simulink model "fw_pos_control"  (R2021a)
settings: Solver=FixedStepAuto  StartTime=0.0  StopTime=5  FixedStep=0.02  RelTol=1e-3
undefined symbols (not defined in the file): DiscIntNeverNeededParam, DT_DEFAULT, FW_AIRSPD_MAX, FW_AIRSPD_MIN, FW_L1_DAMPING, FW_L1_PERIOD, FW_L1_R_SLEW_MAX, FW_R_LIM, FW_T_CLMB_MAX, FW_T_HRATE_FF, FW_T_I_GAIN_PIT, FW_T_I_GAIN_THR, FW_T_PTCH_DAMP, FW_T_RLL2THR, FW_T_SEB_R_FF, FW_T_SINK_MAX, FW_T_SINK_MIN, FW_T_SPD_OMEGA, FW_T_STE_R_TC, FW_T_TAS_TC, FW_T_THR_DAMP, FW_T_VERT_ACC, FW_THR_CRUISE, FW_THR_MAX, FW_THR_MIN, FW_THR_SLEW_MAX, GRAVITY, magnitude
libraries: simulink x28, vrlib x3
(part 3 of 4)

== stateflow chart fw_pos_control/FW Control ==
  state rotary_wing
    en,du:
    sprintf("current sample time is %f", getSimulationTime);
  state fixed_wing
    en,du:
    % 定义中间变量
    fixed_wing.define_variables;
    % 轮询相关数据
    [airspeed_valid_, eas2tas_] = fixed_wing.airspeed_poll;
    [man_ctr_sp_alt_, man_ctr_sp_aspd_] = fixed_wing.manual_control_setpoint_poll;
    [yaw_, pitch_, roll_] = fixed_wing.vehicle_attitude_poll;
    [last_manual_] = fixed_wing.vehicle_control_mode_poll;
    [nav_speed_2d_, ground_speed_2d_] = fixed_wing.vehicle_update_nav_speed;
    % 默认不直接控制方向舵，不使用襟翼，油门不限幅
    out_att_sp.fw_control_yaw = false;
    out_att_sp.apply_flaps = uint8(PX4_VEHICLE_ATTITUDE_SETPOINT.FLAPS_OFF);
    throttle_max_ = 1.0;
    state onGround_or_inTakeoffSituation [parallel]
      settings: executionOrder=1
      state on_ground
        en:
        was_in_air_ = false;
      state in_takeOffSituation
        en:
        %记录起飞时间和起飞高度
        was_in_air_ = true;
        time_went_in_air_ = uint64(getSimulationTime);
        takeoff_ground_alt_ = current_alt_;
        en, du:
        in_takeoff_situation_ = is_takeoff_situation;
      (default) -> on_ground
      on_ground -> in_takeOffSituation : %上一时刻在地上，当前时刻在空中
          | [~was_in_air_ && ~landed_]
      in_takeOffSituation -> on_ground : [landed_]
    state position_control [parallel]
      settings: executionOrder=2
      state mode_select [parallel]
        settings: executionOrder=1
        (default) -> (junction 1468)
        mode_select -> (junction 1468)
        (junction 1468) -> (junction 1469) [order 1] : [control_mode.flag_control_auto_enabled || control_mode.flag_control_offboard_enabled]
        (junction 1468) -> (junction 1470) [order 2]
        (junction 1469) -> (junction 1477) : {pos_control_mode_ = PX4_FW_CONTROL.AUTO_MODE;}
        (junction 1470) -> (junction 1471) [order 1] : [control_mode.flag_control_velocity_enabled && control_mode.flag_control_altitude_enabled]
        (junction 1470) -> (junction 1472) [order 2]
        (junction 1471) -> (junction 1476) : {pos_control_mode_ = PX4_FW_CONTROL.POS_MODE;}
        (junction 1472) -> (junction 1473) [order 1] : [control_mode.flag_control_altitude_enabled]
        (junction 1472) -> (junction 1474) [order 2] : {pos_control_mode_ = PX4_FW_CONTROL.OTHER_MODE;}
        (junction 1473) -> (junction 1475) : {pos_control_mode_ = PX4_FW_CONTROL.ALT_MODE;}
        (junction 1475) -> (junction 1474)
        (junction 1476) -> (junction 1475)
        (junction 1477) -> (junction 1476)
        (junction 1474) -> (junction 1478)
      state mode_action [parallel]
        settings: executionOrder=2
        state auto_offboard_mode [parallel]
          settings: executionOrder=1
          state not_run
            en,du:
          state running
            en,du:
            is_transition_to_fw;
            state auto_logical [parallel]
              settings: executionOrder=1
              (default) -> (junction 2990)
              (junction 2990) -> (junction 2989) [order 1] : [(curr_wp_type_ == PX4_POSITION_SETPOINT.SETPOINT_TYPE_TAKEOFF) && ...
                  |  (~in_takeoff_situation_) && ...
                  |  (airspeed_validated.calibrated_airspeed_m_s >= FW_AIRSPD_MIN)]
              auto_logical -> (junction 2990) : {curr_wp_type_ = uint8(pos_sp_curr_.type);
                  | [dist_xy, dist_z, dist] = get_distance_to_point_global_wgs84(pos_sp_curr_.lat, pos_sp_curr_.lon, pos_sp_curr_.alt, ...
                  |     current_lat_, current_lon_, current_alt_);}
              (junction 2989) -> (junction 2996) : {curr_wp_type_ = uint8(PX4_POSITION_SETPOINT.SETPOINT_TYPE_POSITION);}
              (junction 2990) -> (junction 2992) [order 2]
              (junction 2992) -> (junction 2991) [order 1] : % 飞机还没有越过当前航点，且当前的高度大于2倍FW_CLMBOUT_DIFF，
                  | % 但是水平距离小于2倍可接受的距离以内，飞机改为盘旋的方式靠近当前航点
                  | % FW_CLMBOUT_DIFF 默认10m
                  | [(curr_wp_type_ == PX4_POSITION_SETPOINT.SETPOINT_TYPE_POSITION) && ...
                  |  (dist > 0.0) && ...
                  |  (dist > 2.0 * FW_CLMBOUT_DIFF) && ...
                  |  (dist_xy < 2.0 * max(acc_rad, abs(pos_sp_triplet.current.loiter_radius)))]
              (junction 2991) -> (junction 2995) : {curr_wp_type_ == uint8(PX4_POSITION_SETPOINT.SETPOINT_TYPE_LOITER);}
              (junction 2992) -> (junction 2993) [order 2]
              (junction 2993) -> (junction 2994) [order 1] : % 飞机还没有越过当前航点，且当前的高度大于2倍FW_CLMBOUT_DIFF，
                  | % 同时水平距离也大于2倍可接受的距离以外，飞机继续以position的方式靠近当前航点
                  | % FW_CLMBOUT_DIFF 默认10m
                  | [(curr_wp_type_ == PX4_POSITION_SETPOINT.SETPOINT_TYPE_LOITER) && ...
                  |  (dist > 0.0) && ...
                  |  (dist > 2.0 * FW_CLMBOUT_DIFF) && ...
                  |  (dist_xy < 2.0 * max(acc_rad, max(acc_rad, pos_sp_triplet.current.loiter_radius)))]
              (junction 2993) -> (junction 2997) [order 2]
              (junction 2994) -> (junction 2998) : {curr_wp_type_ == uint8(PX4_POSITION_SETPOINT.SETPOINT_TYPE_POSITION);}
              (junction 2996) -> (junction 2995)
              (junction 2995) -> (junction 2998)
              (junction 2998) -> (junction 2997)
              (junction 2997) -> (junction 2999)
            state auto_action [parallel]
              settings: executionOrder=2
              state idle [parallel]
                settings: executionOrder=1
                state not_run
                  en,du:
                state running
                  en,du:
                  reset_landing_state;
                  reset_takeoff_state(false);
                  out_att_sp.roll_body = single(0.0);
                  out_att_sp.pitch_body = single(deg2rad(FW_PSP_OFF));
                  out_att_sp.thrust_body(1)  = single(0.0);
                  if (was_circle_mode_ && ~circle_mode_)
                  out_att_sp.roll_reset_integral = true;
                  else
                  out_att_sp.roll_reset_integral = false;
                  end
                (default) -> fixed_wing.position_control.mode_action.auto_offboard_mode.running.auto_action.idle.not_run
                fixed_wing.position_control.mode_action.auto_offboard_mode.running.auto_action.idle.not_run -> fixed_wing.position_control.mode_action.auto_offboard_mode.running.auto_action.idle.running : [curr_wp_type_ == uint8(PX4_POSITION_SETPOINT.SETPOINT_TYPE_IDLE)]
                fixed_wing.position_control.mode_action.auto_offboard_mode.running.auto_action.idle.running -> fixed_wing.position_control.mode_action.auto_offboard_mode.running.auto_action.idle.not_run : [curr_wp_type_ ~= uint8(PX4_POSITION_SETPOINT.SETPOINT_TYPE_IDLE)]
              state position [parallel]
                settings: executionOrder=2
                state not_run
                  en,du:
                state running
                  en,du:
                  position_sp_alt = get_foh_alt;
                  % l1控制, 输出att_sp.roll-body, att_sp.yaw_body
                  [out_att_sp.roll_body, out_att_sp.yaw_body, ...
                  l1_target_bearing_, l1_crosstrack_error_, ...
                  l1_distance_, circle_mode_] = ...
                  mode_action.l1_navigate_waypoints(prev_wp_, curr_wp_, curr_pos_, nav_speed_2d_, out_att_sp.roll_body);
                  % tecs控制
                  [run_tecs_, tecs_input_] = mode_action.prepare_tecs_controller_param(position_sp_alt, ...
                  fixed_wing.cal_target_aspd(mission_airspeed_), ...
                  deg2rad(FW_P_LIM_MIN), ...
                  deg2rad(FW_P_LIM_MAX), ...
                  tecs_fw_thr_min, ...
                  tecs_fw_thr_max, ...
                  tecs_fw_mission_throttle, ...
                  false, ...
                  deg2rad(FW_P_LIM_MIN), ...
                  PX4_TECS_STATUS.TECS_MODE_NORMAL, ...
                  nan);
                  % 输出att_sp.pitch_body, roll_reset_integral, thrust_body
                  if (run_tecs_ == true)
                  [tecs_throttle_sp_, tecs_pitch_sp_, tecs_hgt_rate_sp_, tecs_mode_] = mode_action.tecs_controller(tecs_input_);
                  out_att_sp.pitch_body = single(tecs_pitch_sp_ + deg2rad(FW_PSP_OFF));
                  else
                  out_att_sp.pitch_body = single(deg2rad(FW_PSP_OFF));
                  end
                  fixed_wing.reset_landing_state;
                  fixed_wing.reset_takeoff_state(false);
                  if (was_circle_mode_ && ~circle_mode_)
                  out_att_sp.roll_reset_integral = true;
                  else
                  out_att_sp.roll_reset_integral = false;
                  end
                  out_att_sp.thrust_body(1) = constrain(tecs_throttle_sp_, 0.0, 1.0);
                (default) -> fixed_wing.position_control.mode_action.auto_offboard_mode.running.auto_action.position.not_run
                fixed_wing.position_control.mode_action.auto_offboard_mode.running.auto_action.position.not_run -> fixed_wing.position_control.mode_action.auto_offboard_mode.running.auto_action.position.running : [curr_wp_type_ == uint8(PX4_POSITION_SETPOINT.SETPOINT_TYPE_POSITION)]
                fixed_wing.position_control.mode_action.auto_offboard_mode.running.auto_action.position.running -> fixed_wing.position_control.mode_action.auto_offboard_mode.running.auto_action.position.not_run : [curr_wp_type_ ~= uint8(PX4_POSITION_SETPOINT.SETPOINT_TYPE_POSITION)]
              state loiter [parallel]
                settings: executionOrder=3
                state not_run
                  en,du:
                state running
                  en,du:
                  [out_att_sp.roll_body, out_att_sp.yaw_body, l1_target_bearing_, l1_distance_, circle_mode_] = ...
                  mode_action.l1_navigate_loiter(curr_wp_, curr_pos_, ...
                  pos_sp_curr_.loiter_direction, nav_speed_2d_, ...
                  pos_sp_curr_.loiter_radius, circle_mode_, out_att_sp.roll_body);
                  state loiter_logical [parallel]
                    settings: executionOrder=1
                    (default) -> (junction 3043)
                    (junction 3043) -> (junction 3044) [order 1] : [pos_sp_triplet.next.type == PX4_POSITION_SETPOINT.SETPOINT_TYPE_LAND && ...
                        | pos_sp_triplet.next.valid && ...
                        | circle_mode_ && ...
                        | FW_LND_EARLYCFG]
                    (junction 3043) -> (junction 3045) [order 2]
                    (junction 3044) -> (junction 3052) : {loiter_type_ = PX4_LOITER_TYPE.NEXT_WP_LAND}
                    (junction 3045) -> (junction 3046) [order 1] : [in_takeoff_situation_]
                    (junction 3045) -> (junction 3047) [order 2]
                    (junction 3046) -> (junction 3051) : {loiter_type_ = PX4_LOITER_TYPE.IN_TAKEOFF_SITUATION}
                    (junction 3047) -> (junction 3048) [order 1] : [land_abort_]
                    (junction 3047) -> (junction 3049) [order 2] : {loiter_type_ = PX4_LOITER_TYPE.DEFAULT}
                    (junction 3048) -> (junction 3050) : {loiter_type_ = PX4_LOITER_TYPE.LAND_ABORT}
                    (junction 3050) -> (junction 3049)
                    (junction 3051) -> (junction 3050)
                    (junction 3052) -> (junction 3051)
                    (junction 3049) -> (junction 3053)
                  state loiter_action [parallel]
                    settings: executionOrder=2
                    state next_wp_land [parallel]
                      settings: executionOrder=1
                      state not_run
                        en,du:
                      state running
                        en,du:
                        tecs_height_error_gain_ = single(1.0 / max(FW_LND_THRTC_SC * FW_T_ALT_TC, 0.1));
                        out_att_sp.apply_flaps = uint8(PX4_VEHICLE_ATTITUDE_SETPOINT.FLAPS_LAND);
                        [run_tecs_, tecs_input_] = mode_action.prepare_tecs_controller_param(pos_sp_curr_.alt, ...
                        fixed_wing.cal_target_aspd(FW_LND_AIRSPD_SC * FW_AIRSPD_MIN), ...
                        deg2rad(FW_P_LIM_MIN), ...
                        deg2rad(FW_P_LIM_MAX), ...
                        tecs_fw_thr_min, ...
                        tecs_fw_thr_max, ...
                        tecs_fw_mission_throttle, ...
                        false, ...
                        deg2rad(FW_P_LIM_MIN), ...
                        PX4_TECS_STATUS.TECS_MODE_NORMAL, ...
                        nan);
                        if (run_tecs_ == true)
                        [tecs_throttle_sp_, tecs_pitch_sp_, tecs_hgt_rate_sp_, tecs_mode_] = ...
                        mode_action.tecs_controller(tecs_input_);
                        out_att_sp.pitch_body = single(tecs_pitch_sp_ + deg2rad(FW_PSP_OFF));
                        else
                        out_att_sp.pitch_body = single(deg2rad(FW_PSP_OFF));
                        end
                        fixed_wing.reset_landing_state;
                        fixed_wing.reset_takeoff_state(false);
                        if (was_circle_mode_ && ~circle_mode_)
                        out_att_sp.roll_reset_integral = true;
                        else
                        out_att_sp.roll_reset_integral = true;
                        end
                        out_att_sp.thrust_body(1) = tecs_throttle_sp_;
                      (default) -> fixed_wing.position_control.mode_action.auto_offboard_mode.running.auto_action.loiter.running.loiter_action.next_wp_land.not_run
                      fixed_wing.position_control.mode_action.auto_offboard_mode.running.auto_action.loiter.running.loiter_action.next_wp_land.not_run -> fixed_wing.position_control.mode_action.auto_offboard_mode.running.auto_action.loiter.running.loiter_action.next_wp_land.running : [loiter_type_ == PX4_LOITER_TYPE.NEXT_WP_LAND]
                      fixed_wing.position_control.mode_action.auto_offboard_mode.running.auto_action.loiter.running.loiter_action.next_wp_land.running -> fixed_wing.position_control.mode_action.auto_offboard_mode.running.auto_action.loiter.running.loiter_action.next_wp_land.not_run : [loiter_type_ ~= PX4_LOITER_TYPE.NEXT_WP_LAND]
                    state in_takeoff_situation [parallel]
                      settings: executionOrder=2
                      state runing
                        en,du:
                        out_att_sp.roll_body = constrain(out_att_sp.roll_body, deg2rad(-5.0), deg2rad(5.0));
                        [run_tecs_, tecs_input_] = mode_action.prepare_tecs_controller_param(...
                        max(pos_sp_curr_.alt, takeoff_ground_alt_ + FW_CLMBOUT_DIFF), ...
                        cal_target_aspd(mission_airspeed_), ...
                        deg2rad(FW_P_LIM_MIN), ...
                        deg2rad(FW_P_LIM_MAX), ...
                        tecs_fw_thr_min, ...
                        tecs_fw_thr_max, ...
                        tecs_fw_mission_throttle, ...
                        false, ...
                        deg2rad(FW_P_LIM_MIN), ...
                        PX4_TECS_STATUS.TECS_MODE_NORMAL, ...
                        nan);
                        if (run_tecs_ == true)
                        [tecs_throttle_sp_, tecs_pitch_sp_, tecs_hgt_rate_sp_, tecs_mode_] = tecs_controller(tecs_input_);
                        out_att_sp.pitch_body = single(tecs_pitch_sp_ + deg2rad(FW_PSP_OFF));
                        else
                        out_att_sp.pitch_body = single(deg2rad(FW_PSP_OFF));
                        end
                        fixed_wing.reset_landing_state;
                        fixed_wing.reset_takeoff_state(false);
                        if (was_circle_mode_ && ~circle_mode_)
                        out_att_sp.roll_reset_integral = true;
                        end
                        out_att_sp.thrust_body(1) = tecs_throttle_sp_;
                      state not_run
                        en,du:
                      (default) -> fixed_wing.position_control.mode_action.auto_offboard_mode.running.auto_action.loiter.running.loiter_action.in_takeoff_situation.not_run
                      fixed_wing.position_control.mode_action.auto_offboard_mode.running.auto_action.loiter.running.loiter_action.in_takeoff_situation.not_run -> runing : [loiter_type_ == PX4_LOITER_TYPE.IN_TAKEOFF_SITUATION]
                      runing -> fixed_wing.position_control.mode_action.auto_offboard_mode.running.auto_action.loiter.running.loiter_action.in_takeoff_situation.not_run : [loiter_type_ ~= PX4_LOITER_TYPE.IN_TAKEOFF_SITUATION]
                    state land_abort [parallel]
                      settings: executionOrder=3
                      state running
                        en,du:
                        % aborted landing complete, normal loiter over landing point
                        if (pos_sp_curr_.alt - current_alt_ < FW_CLMBOUT_DIFF)
                        land_abort_ = false;
                        else
                        % continue straight until vehicle has sufficient altitude
                        out_att_sp.roll_body = single(0.0);
                        end
                        tecs_height_error_gain_ = single(1.0 / max(FW_LND_THRTC_SC * FW_T_ALT_TC, 0.1));
                        [run_tecs_, tecs_input_] = mode_action.prepare_tecs_controller_param(pos_sp_curr_.alt, ...
                        cal_target_aspd(mission_airspeed_), ...
                        deg2rad(FW_P_LIM_MIN), ...
                        deg2rad(FW_P_LIM_MAX), ...
                        tecs_fw_thr_min, ...
                        tecs_fw_thr_max, ...
                        tecs_fw_mission_throttle, ...
                        false, ...
                        deg2rad(FW_P_LIM_MIN), ...
                        PX4_TECS_STATUS.TECS_MODE_NORMAL, ...
                        nan);
                        if (run_tecs_ == true)
                        [tecs_throttle_sp_, tecs_pitch_sp_, tecs_hgt_rate_sp_, tecs_mode_] = mode_action.tecs_controller(tecs_input_);
                        out_att_sp.pitch_body = single(tecs_pitch_sp_ + deg2rad(FW_PSP_OFF));
                        else
                        out_att_sp.pitch_body = single(deg2rad(FW_PSP_OFF));
                        end
                        fixed_wing.reset_landing_state;
                        fixed_wing.reset_takeoff_state(false);
                        if (was_circle_mode_ && ~circle_mode_)
                        out_att_sp.roll_reset_integral = true;
                        else
                        out_att_sp.roll_reset_integral = false;
                        end
                        out_att_sp.thrust_body(1) = tecs_throttle_sp_;
                      state not_run
                        en,du:
                      (default) -> fixed_wing.position_control.mode_action.auto_offboard_mode.running.auto_action.loiter.running.loiter_action.land_abort.not_run
                      fixed_wing.position_control.mode_action.auto_offboard_mode.running.auto_action.loiter.running.loiter_action.land_abort.not_run -> fixed_wing.position_control.mode_action.auto_offboard_mode.running.auto_action.loiter.running.loiter_action.land_abort.running : [loiter_type_ == PX4_LOITER_TYPE.LAND_ABORT]
                      fixed_wing.position_control.mode_action.auto_offboard_mode.running.auto_action.loiter.running.loiter_action.land_abort.running -> fixed_wing.position_control.mode_action.auto_offboard_mode.running.auto_action.loiter.running.loiter_action.land_abort.not_run : [loiter_type_ ~= PX4_LOITER_TYPE.LAND_ABORT]
                    state default [parallel]
                      settings: executionOrder=4
                      state not_run
                        en,du:
                      state running
                        en,du:
                        [run_tecs_, tecs_input_] = mode_action.prepare_tecs_controller_param(pos_sp_curr_.alt, ...
                        airspeed_demand_, ...
                        deg2rad(FW_P_LIM_MIN), ...
                        deg2rad(FW_P_LIM_MAX), ...
                        tecs_fw_thr_min, ...
                        tecs_fw_thr_max, ...
                        tecs_fw_mission_throttle, ...
                        false, ...
                        deg2rad(FW_P_LIM_MIN), ...
                        PX4_TECS_STATUS.TECS_MODE_NORMAL, ...
                        nan);
                        if (run_tecs_ == true)
                        [tecs_throttle_sp_, tecs_pitch_sp_, tecs_hgt_rate_sp_, tecs_mode_] = mode_action.tecs_controller(tecs_input_);
                        out_att_sp.pitch_body = single(tecs_pitch_sp_ + deg2rad(FW_PSP_OFF));
                        else
                        out_att_sp.pitch_body = single(deg2rad(FW_PSP_OFF));
                        end
                        fixed_wing.reset_landing_state;
                        fixed_wing.reset_takeoff_state(false);
                        if (was_circle_mode_ && ~circle_mode_)
                        out_att_sp.roll_reset_integral = true;
                        else
                        out_att_sp.roll_reset_integral = false;
                        end
                        out_att_sp.thrust_body(1) = tecs_throttle_sp_;
                      (default) -> fixed_wing.position_control.mode_action.auto_offboard_mode.running.auto_action.loiter.running.loiter_action.default.not_run
                      fixed_wing.position_control.mode_action.auto_offboard_mode.running.auto_action.loiter.running.loiter_action.default.not_run -> fixed_wing.position_control.mode_action.auto_offboard_mode.running.auto_action.loiter.running.loiter_action.default.running : [loiter_type_ == PX4_LOITER_TYPE.DEFAULT]
                      fixed_wing.position_control.mode_action.auto_offboard_mode.running.auto_action.loiter.running.loiter_action.default.running -> fixed_wing.position_control.mode_action.auto_offboard_mode.running.auto_action.loiter.running.loiter_action.default.not_run : [loiter_type_ ~= PX4_LOITER_TYPE.DEFAULT]
                (default) -> fixed_wing.position_control.mode_action.auto_offboard_mode.running.auto_action.loiter.not_run
                fixed_wing.position_control.mode_action.auto_offboard_mode.running.auto_action.loiter.not_run -> fixed_wing.position_control.mode_action.auto_offboard_mode.running.auto_action.loiter.running : [curr_wp_type_ == uint8(PX4_POSITION_SETPOINT.SETPOINT_TYPE_LOITER)]
                fixed_wing.position_control.mode_action.auto_offboard_mode.running.auto_action.loiter.running -> fixed_wing.position_control.mode_action.auto_offboard_mode.running.auto_action.loiter.not_run : [curr_wp_type_ ~= uint8(PX4_POSITION_SETPOINT.SETPOINT_TYPE_LOITER)]
              state landing [parallel]
                settings: executionOrder=4
                state not_run
                  en,du:
                state running
                  en:
                  fixed_wing.reset_landing_state;
                  time_started_landing_ = uint64(getSimulationTime);
                  en,du:
                  control_landing;
                  land_terrain_alt_ = pos_sp_curr_.alt;
                  out_att_sp.apply_flaps = uint8(PX4_VEHICLE_ATTITUDE_SETPOINT.FLAPS_LAND);
                  state horizontal_control [parallel]
                    settings: executionOrder=1
                    state normal_navigation
                      en,du:
                      [out_att_sp.roll_body, out_att_sp.yaw_body, ...
                      l1_target_bearing_, l1_crosstrack_error_, ...
                      l1_distance_, circle_mode_] = ...
                      mode_action.l1_navigate_waypoints(prev_wp_, ...
                      curr_wp_, curr_pos_, ...
                      nav_speed_2d_, ...
                      out_att_sp.roll_body);
                    state heading_hold
                      en,du:
                      if (pos_sp_prev_.valid)
                      target_bearing_ = bearing_lastwp_currwp_;
                      else
                      target_bearing_ = yaw_;
                      end
                      land_noreturn_horizontal_ = true;
                      [out_att_sp.roll_body, circle_mode_, l1_distance_] = ...
                      mode_action.l1_navigate_heading(target_bearing_, yaw_, ...
                      nav_speed_2d_, out_att_sp.roll_body);
                      out_att_sp.roll_body = constrain(out_att_sp.roll_body, ...
                      deg2rad(10.0), deg2rad(-10.0));
                    (default) -> normal_navigation
                    normal_navigation -> heading_hold : % FW_LND_HHDIST: Landing heading hold horizontal distance, 15m
                        | [(FW_LND_HHDIST > 0.0) && ...
                        |  (~land_noreturn_horizontal_) &&...
                        |  (wp_distance_ < FW_LND_HHDIST) || ...
                        |  (land_noreturn_vertical_)]
                  state vertical_control [parallel]
                    settings: executionOrder=2
                    state glide_slope
                      en,du:
                      [run_tecs_, tecs_input_] = mode_action.prepare_tecs_controller_param(glide_slope, ...
                      cal_target_aspd(FW_LND_AIRSPD_SC * FW_AIRSPD_MIN), ...
                      deg2rad(FW_P_LIM_MIN), ...
                      deg2rad(FW_P_LIM_MAX), ...
                      FW_THR_MIN, ...
                      FW_THR_MAX, ...
                      FW_THR_CRUISE, ...
                      false, ...
                      deg2rad(FW_P_LIM_MIN), ...
                      PX4_TECS_STATUS.TECS_MODE_NORMAL, ...
                      nan);
                      if (run_tecs_ == true)
                      [tecs_throttle_sp_, tecs_pitch_sp_, tecs_hgt_rate_sp_, tecs_mode_] = tecs_controller(tecs_input_);
                      out_att_sp.pitch_body = single(tecs_pitch_sp_ + deg2rad(FW_PSP_OFF));
                      else
                      out_att_sp.pitch_body = single(deg2rad(FW_PSP_OFF));
                      end
                      fixed_wing.reset_takeoff_state(false);
                      if (was_circle_mode_ && ~circle_mode_)
                      out_att_sp.roll_reset_integral = true;
                      end
                    state start_flaring
                      en,du:
                      [land_tecs_mode, land_climbout_pitch_min_rad] = start_flaring;
                      [run_tecs_, tecs_input_] = mode_action.prepare_tecs_controller_param(land_terrain_alt_, ...
                      cal_target_aspd(FW_LND_AIRSPD_SC * FW_AIRSPD_MIN), ...
                      deg2rad(FW_P_LIM_MIN), ...
                      deg2rad(FW_P_LIM_MAX), ...
                      tecs_fw_thr_min, ...
                      tecs_fw_thr_max, ...
                      tecs_fw_mission_throttle, ...
                      false, ...
                      land_climbout_pitch_min_rad, ...
                      land_tecs_mode, ...
                      nan);
                      if (run_tecs_ == true)
                      [tecs_throttle_sp_, tecs_pitch_sp_, tecs_hgt_rate_sp_, tecs_mode_] = tecs_controller(tecs_input_);
                      out_att_sp.pitch_body = single(tecs_pitch_sp_ + deg2rad(FW_PSP_OFF));
                      else
                      out_att_sp.pitch_body = single(deg2rad(FW_PSP_OFF));
                      end
                      if (~land_noreturn_vertical_)
                      % 进入拉平阶段
                      flare_pitch_sp = single(deg2rad(FW_PSP_OFF));
                      flare_height = current_alt_ - land_terrain_alt_;
                      land_noreturn_vertical_ = true;
                      elseif (local_pos.vz > 0.1)
                      % otherwise continue using previous _flare_pitch_sp
                      flare_pitch_sp = single(deg2rad(FW_LND_FL_PMIN) * ...
                      constrain((flare_height - (current_alt_ - land_terrain_alt_)) / flare_height, 0.0, 1.0));
                      end
                      out_att_sp.pitch_body   = flare_pitch_sp;
                      flare_curve_alt_rel_last = flare_curve_alt_rel;
                      fixed_wing.reset_takeoff_state(false);
                      if (was_circle_mode_ && ~circle_mode_)
                      out_att_sp.roll_reset_integral = true;
                      end
                    (default) -> glide_slope
                    glide_slope -> start_flaring : [(current_alt_ < land_terrain_alt_ + ...
                        | flare_curve_alt_rel) || ...
                        | land_noreturn_vertical_]
                (default) -> fixed_wing.position_control.mode_action.auto_offboard_mode.running.auto_action.landing.not_run
                fixed_wing.position_control.mode_action.auto_offboard_mode.running.auto_action.landing.not_run -> fixed_wing.position_control.mode_action.auto_offboard_mode.running.auto_action.landing.running : [curr_wp_type_ == uint8(PX4_POSITION_SETPOINT.SETPOINT_TYPE_LAND)]
                fixed_wing.position_control.mode_action.auto_offboard_mode.running.auto_action.landing.running -> fixed_wing.position_control.mode_action.auto_offboard_mode.running.auto_action.landing.not_run : [curr_wp_type_ ~= uint8(PX4_POSITION_SETPOINT.SETPOINT_TYPE_LAND)]
              state takeoff [parallel]
                settings: executionOrder=5
                state not_run
                  en,du:
                state running
                  en,du:
                  out_att_sp.apply_flaps = uint8(PX4_VEHICLE_ATTITUDE_SETPOINT.FLAPS_TAKEOFF);
                  state other_takeoff_methods
                    en,du:
                  state runway_takeoff
                    en:
                    takeoff_init;
                    en,du:
                    takeoff_terrain_alt_ = get_terrain_altitude_takeoff;
                    % l1控制, 输出att_sp.roll-body, att_sp.yaw_body
                    [takeoff_roll_body_, takeoff_yaw_body_, ...
                    l1_target_bearing_, l1_crosstrack_error_, ...
                    l1_distance_, circle_mode_] = ...
                    mode_action.l1_navigate_waypoints(prev_wp_, curr_wp_, curr_pos_, nav_speed_2d_, out_att_sp.roll_body);
                    % prepare tecs controller data
                    [airspeed, alt_agl] = cal_airspeed_alt(takeoff_terrain_alt_);
                    if (RWTO_MAX_PITCH > 0.1)
                    takeoff_pitch_max_deg_ = RWTO_MAX_PITCH;
                    else
                    takeoff_pitch_max_deg_ = FW_P_LIM_MAX;
                    end
                    state throttle_ramp
                      en,du:
                      ramp_time_ = uint64(getSimulationTime) - takeoff_initialized_time_;
                      [run_tecs_, tecs_input_] = prepare_tecs_controller_param(pos_sp_curr_.alt, ...
                      cal_target_aspd(RWTO_AIRSPD_SCL * FW_AIRSPD_MIN), ...
                      deg2rad(FW_P_LIM_MIN), ...
                      deg2rad(takeoff_pitch_max_deg_), ...
                      FW_THR_MIN, ...
                      FW_THR_MAX, ...
                      FW_THR_CRUISE, ...
                      takeoff_climbout_, ...
                      deg2rad(FW_TKO_PITCH_MIN), ...
                      PX4_TECS_STATUS.TECS_MODE_TAKEOFF, ...
                      nan);
                      if (run_tecs_ == true)
                      [tecs_throttle_sp_, tecs_pitch_sp_, tecs_hgt_rate_sp_, tecs_mode_] = tecs_controller(tecs_input_);
                      out_att_sp.pitch_body = single(tecs_pitch_sp_ + deg2rad(FW_PSP_OFF));
                      else
                      out_att_sp.pitch_body = single(deg2rad(FW_PSP_OFF));
                      end
                      % 输出att_sp
                      out_att_sp.roll_body = single(0.0);
                      if (RWTO_HDG == single(0))
                      out_att_sp.yaw_body = takeoff_init_yaw_;
                      else
                      out_att_sp.yaw_body = takeoff_yaw_body_;
                      end
                      out_att_sp.fw_control_yaw = true;
                      out_att_sp.pitch_body = single(deg2rad(RWTO_PSP));
                      out_att_sp.roll_reset_integral = true;
                      out_att_sp.pitch_reset_integral = true;
                      fixed_wing.reset_landing_state;
                      if (was_circle_mode_ && ~circle_mode_)
                      out_att_sp.roll_reset_integral = true;
                      end
                      out_att_sp.thrust_body(1) = min(single(double(ramp_time_) / (RWTO_RAMP_TIME * 1000) * ...
                      RWTO_MAX_THR), RWTO_MAX_THR);
                    state clamped_to_runway
                      en,du:
                      [run_tecs_, tecs_input_] = prepare_tecs_controller_param(pos_sp_curr_.alt, ...
                      cal_target_aspd(RWTO_AIRSPD_SCL * FW_AIRSPD_MIN), ...
                      deg2rad(FW_P_LIM_MIN), ...
                      deg2rad(takeoff_pitch_max_deg_), ...
                      FW_THR_MIN, ...
                      FW_THR_MAX, ...
                      FW_THR_CRUISE, ...
                      takeoff_climbout_, ...
                      deg2rad(FW_TKO_PITCH_MIN), ...
                      PX4_TECS_STATUS.TECS_MODE_TAKEOFF, ...
                      nan);
                      if (run_tecs_ == true)
                      [tecs_throttle_sp_, tecs_pitch_sp_, tecs_hgt_rate_sp_, tecs_mode_] = tecs_controller(tecs_input_);
                      out_att_sp.pitch_body = single(tecs_pitch_sp_ + deg2rad(FW_PSP_OFF));
                      else
                      out_att_sp.pitch_body = single(deg2rad(FW_PSP_OFF));
                      end
                      % 输出att_sp
                      out_att_sp.roll_body = single(0.0);
                      if (RWTO_HDG == single(0))
                      out_att_sp.yaw_body = takeoff_init_yaw_;
                      else
                      out_att_sp.yaw_body = takeoff_yaw_body_;
                      end
                      out_att_sp.fw_control_yaw = true;
                      out_att_sp.pitch_body = single(deg2rad(RWTO_PSP));
                      out_att_sp.roll_reset_integral = true;
                      out_att_sp.pitch_reset_integral = true;
                      fixed_wing.reset_landing_state;
                      if (was_circle_mode_ && ~circle_mode_)
                      out_att_sp.roll_reset_integral = true;
                      end
                      out_att_sp.thrust_body(1) = RWTO_MAX_THR;
                    state takeoff
                      en,du:
                      [run_tecs_, tecs_input_] = prepare_tecs_controller_param(pos_sp_curr_.alt, ...
                      cal_target_aspd(RWTO_AIRSPD_SCL * FW_AIRSPD_MIN), ...
                      deg2rad(FW_P_LIM_MIN), ...
                      deg2rad(takeoff_pitch_max_deg_), ...
                      FW_THR_MIN, ...
                      FW_THR_MAX, ...
                      FW_THR_CRUISE, ...
                      takeoff_climbout_, ...
                      deg2rad(FW_TKO_PITCH_MIN), ...
                      PX4_TECS_STATUS.TECS_MODE_TAKEOFF, ...
                      nan);
                      if (run_tecs_ == true)
                      [tecs_throttle_sp_, tecs_pitch_sp_, tecs_hgt_rate_sp_, tecs_mode_] = tecs_controller(tecs_input_);
                      out_att_sp.pitch_body = single(tecs_pitch_sp_ + deg2rad(FW_PSP_OFF));
                      else
                      out_att_sp.pitch_body = single(deg2rad(FW_PSP_OFF));
                      end
                      % 输出att_sp
                      out_att_sp.roll_body = single(0.0);
                      if (RWTO_HDG == single(0))
                      out_att_sp.yaw_body = takeoff_init_yaw_;
                      else
                      out_att_sp.yaw_body = takeoff_yaw_body_;
                      end
                      out_att_sp.fw_control_yaw = true;
                      out_att_sp.pitch_body = tecs_pitch_sp_;
                      out_att_sp.roll_reset_integral = false;
                      out_att_sp.pitch_reset_integral = false;
                      fixed_wing.reset_landing_state;
                      if (was_circle_mode_ && ~circle_mode_)
                      out_att_sp.roll_reset_integral = true;
                      end
                      out_att_sp.thrust_body(1) = tecs_throttle_sp_;
                    state climbout
                      en,du:
                      [run_tecs_, tecs_input_] = prepare_tecs_controller_param(pos_sp_curr_.alt, ...
                      cal_target_aspd(RWTO_AIRSPD_SCL * FW_AIRSPD_MIN), ...
                      deg2rad(FW_P_LIM_MIN), ...
                      deg2rad(takeoff_pitch_max_deg_), ...
                      FW_THR_MIN, ...
                      FW_THR_MAX, ...
                      FW_THR_CRUISE, ...
                      takeoff_climbout_, ...
                      deg2rad(FW_TKO_PITCH_MIN), ...
                      PX4_TECS_STATUS.TECS_MODE_TAKEOFF, ...
                      nan);
                      if (run_tecs_ == true)
                      [tecs_throttle_sp_, tecs_pitch_sp_, tecs_hgt_rate_sp_, tecs_mode_] = tecs_controller(tecs_input_);
                      out_att_sp.pitch_body = single(tecs_pitch_sp_ + deg2rad(FW_PSP_OFF));
                      else
                      out_att_sp.pitch_body = single(deg2rad(FW_PSP_OFF));
                      end
                      % 输出att_sp
                      out_att_sp.roll_body = constrain(takeoff_roll_body_, -RWTO_MAX_ROLL, RWTO_MAX_ROLL);
                      if (RWTO_HDG == single(0))
                      out_att_sp.yaw_body = takeoff_init_yaw_;
                      else
                      out_att_sp.yaw_body = takeoff_yaw_body_;
                      end
                      out_att_sp.fw_control_yaw = false;
                      out_att_sp.pitch_body = tecs_pitch_sp_;
                      out_att_sp.roll_reset_integral = false;
                      out_att_sp.pitch_reset_integral = false;
                      fixed_wing.reset_landing_state;
                      if (was_circle_mode_ && ~circle_mode_)
                      out_att_sp.roll_reset_integral = true;
                      end
                      out_att_sp.thrust_body(1) = tecs_throttle_sp_;
                    (default) -> throttle_ramp
                    fixed_wing.position_control.mode_action.auto_offboard_mode.running.auto_action.takeoff.running.runway_takeoff.takeoff -> climbout : [alt_agl > FW_CLMBOUT_DIFF]
                    throttle_ramp -> clamped_to_runway : [(ramp_time_ > RWTO_RAMP_TIME * 1000) || ...
                        | (airspeed > FW_AIRSPD_MIN * RWTO_AIRSPD_SCL * 0.9)]
                    clamped_to_runway -> fixed_wing.position_control.mode_action.auto_offboard_mode.running.auto_action.takeoff.running.runway_takeoff.takeoff : [airspeed > FW_AIRSPD_MIN * RWTO_AIRSPD_SCL]
                  (default) -> other_takeoff_methods
                  other_takeoff_methods -> runway_takeoff : % 滑跑起飞
                      | [RWTO_TKOFF]
                  runway_takeoff -> other_takeoff_methods : [~RWTO_TKOFF]
                (default) -> fixed_wing.position_control.mode_action.auto_offboard_mode.running.auto_action.takeoff.not_run
                fixed_wing.position_control.mode_action.auto_offboard_mode.running.auto_action.takeoff.not_run -> fixed_wing.position_control.mode_action.auto_offboard_mode.running.auto_action.takeoff.running : [curr_wp_type_ == uint8(PX4_POSITION_SETPOINT.SETPOINT_TYPE_TAKEOFF)]
                fixed_wing.position_control.mode_action.auto_offboard_mode.running.auto_action.takeoff.running -> fixed_wing.position_control.mode_action.auto_offboard_mode.running.auto_action.takeoff.not_run : [curr_wp_type_ ~= uint8(PX4_POSITION_SETPOINT.SETPOINT_TYPE_TAKEOFF)]
          (default) -> fixed_wing.position_control.mode_action.auto_offboard_mode.not_run
          fixed_wing.position_control.mode_action.auto_offboard_mode.not_run -> fixed_wing.position_control.mode_action.auto_offboard_mode.running : [pos_control_mode_ == PX4_FW_CONTROL.AUTO_MODE]
          fixed_wing.position_control.mode_action.auto_offboard_mode.running -> fixed_wing.position_control.mode_action.auto_offboard_mode.not_run : [pos_control_mode_ ~= PX4_FW_CONTROL.AUTO_MODE]
        state pos_mode [parallel]
          settings: executionOrder=2
          state not_run
            en,du:
          state running
            en:
            % Need to init because last loop iteration was in a different mode
            pos_mode_hold_alt_ = current_alt_;
            hdg_hold_yaw = yaw_;
            % reset setpoints from other modes (auto) otherwise we won't level out without new manual input
            out_att_sp.roll_body = single(man_ctr_sp.y * deg2rad(FW_MAN_R_MAX));
            out_att_sp.yaw_body = single(0.0);
            en,du:
            pos_mode_altctrl_airspeed = mode_action.get_demanded_airspeed;
            pos_mode_desire_alt = mode_action.update_desired_altitude;
            [pos_mode_hold_alt_, pos_mode_pitch_limited_min_, pos_mode_throttle_max_] = mode_action.do_takeoff_help;
            [run_tecs_, tecs_input_] = mode_action.prepare_tecs_controller_param(pos_mode_desire_alt, ...
            pos_mode_altctrl_airspeed, ...
            deg2rad(FW_P_LIM_MIN), ...
            deg2rad(FW_P_LIM_MAX), ...
            FW_THR_MIN, ...
            tecs_fw_thr_max, ...
            tecs_fw_mission_throttle, ...
            false, ...
            deg2rad(FW_P_LIM_MIN), ...
            PX4_TECS_STATUS.TECS_MODE_NORMAL, ...
            manual_height_rate_setpoint_m_s_);
            if (run_tecs_ == true)
            [tecs_throttle_sp_, tecs_pitch_sp_, tecs_hgt_rate_sp_, tecs_mode_] = tecs_controller(tecs_input_);
            out_att_sp.pitch_body = single(tecs_pitch_sp_ + deg2rad(FW_PSP_OFF));
            else
            out_att_sp.pitch_body = single(deg2rad(FW_PSP_OFF));
            end
            heading_control(pos_mode_hold_alt_);
            out_att_sp.thrust_body(1) = tecs_throttle_sp_;
          (default) -> fixed_wing.position_control.mode_action.pos_mode.not_run
          fixed_wing.position_control.mode_action.pos_mode.not_run -> fixed_wing.position_control.mode_action.pos_mode.running : [pos_control_mode_ == PX4_FW_CONTROL.POS_MODE]
          fixed_wing.position_control.mode_action.pos_mode.running -> fixed_wing.position_control.mode_action.pos_mode.not_run : [pos_control_mode_ ~= PX4_FW_CONTROL.POS_MODE]
        state [roll_body,nav_bearing,target_braring,crosstrack_error, ... [function]
          distance,circle_mode] = l1_navigate_waypoints(vector_A, ...
          vector_B,vector_curr_position,ground_speed_vector,att_sp_roll_body)
        state [roll_sp,circle_mode,l1_heading_dis] = ... [function]
          l1_navigate_heading(navigation_heading,current_heading,...
          ground_speed_vector,att_sp_roll_body)
        state [roll_sp,nav_bearing,target_bearing,distance,circle_mode] = ... [function]
          l1_navigate_loiter(vector_A,vector_curr_position, ...
          loiter_direction,ground_speed_vector,radius,curr_circle_mode,att_sp_roll_body)
        state [throttle_sp,pitch_sp,hgt_rate_sp,tecs_mode] = tecs_controller(tecs_input) [function]
        state alt_mode [parallel]
          settings: executionOrder=3
          state not_run
            en,du:
          state running
            % 高度控制: pitch stick moves altitude setpoint, throttle stick sets airspeed
            en:
            alt_mode_alt_hold = current_alt_;
            en,du:
            alt_mode_altctrl_airspeed = mode_action.get_demanded_airspeed;
            alt_mode_desire_alt = mode_action.update_desired_altitude;
            [run_tecs_, tecs_input_] = mode_action.prepare_tecs_controller_param(alt_mode_desire_alt, ...
            alt_mode_altctrl_airspeed, ...
            deg2rad(FW_P_LIM_MIN), ...
            deg2rad(FW_P_LIM_MAX), ...
            FW_THR_MIN, ...
            tecs_fw_thr_max, ...
            tecs_fw_mission_throttle, ...
            false, ...
            deg2rad(FW_P_LIM_MIN), ...
            PX4_TECS_STATUS.TECS_MODE_NORMAL, ...
            manual_height_rate_setpoint_m_s_);
            if (run_tecs_ == true)
            [tecs_throttle_sp_, tecs_pitch_sp_, tecs_hgt_rate_sp_, tecs_mode_] = tecs_controller(tecs_input_);
            out_att_sp.pitch_body = single(tecs_pitch_sp_ + deg2rad(FW_PSP_OFF));
            else
            out_att_sp.pitch_body = single(deg2rad(FW_PSP_OFF));
            end
            out_att_sp.roll_body = single(man_ctr_sp.y * deg2rad(FW_MAN_R_MAX));
            out_att_sp.yaw_body = single(0.0);
            out_att_sp.thrust_body(1) = tecs_throttle_sp_;
          (default) -> fixed_wing.position_control.mode_action.alt_mode.not_run
          fixed_wing.position_control.mode_action.alt_mode.not_run -> fixed_wing.position_control.mode_action.alt_mode.running : [pos_control_mode_ == PX4_FW_CONTROL.ALT_MODE]
          fixed_wing.position_control.mode_action.alt_mode.running -> fixed_wing.position_control.mode_action.alt_mode.not_run : [pos_control_mode_ ~= PX4_FW_CONTROL.ALT_MODE]
        state other_mode [parallel]
          settings: executionOrder=4
          state not_run
            en,du:
          state running
            en,du:
            other_mode_alt_hold = current_alt_;
            % 重置tecs状态
            reinitialize_tecs_ = false;
            % reset landing and takeoff state
            if (~last_manual_)
            fixed_wing.reset_landing_state();
            fixed_wing.reset_takeoff_state(false);
            end
            out_att_sp.thrust_body(1) = min(out_att_sp.thrust_body(1), RWTO_MAX_THR);
          (default) -> fixed_wing.position_control.mode_action.other_mode.not_run
          fixed_wing.position_control.mode_action.other_mode.not_run -> fixed_wing.position_control.mode_action.other_mode.running : [pos_control_mode_ == PX4_FW_CONTROL.OTHER_MODE]
          fixed_wing.position_control.mode_action.other_mode.running -> fixed_wing.position_control.mode_action.other_mode.not_run : [pos_control_mode_ ~= PX4_FW_CONTROL.OTHER_MODE]
      state pub_pos_ctrl_status [parallel]
        % 后续可以将att_sp的topic放在这里发布
        en,du:
        pos_ctrl_status.timestamp = uint64(getSimulationTime);
        pos_ctrl_status.type = curr_wp_type_;
        pos_ctrl_status.nav_roll = out_att_sp.roll_body;
        pos_ctrl_status.nav_pitch = out_att_sp.pitch_body;
        pos_ctrl_status.nav_bearing = l1_target_bearing_;
        pos_ctrl_status.target_bearing = l1_target_bearing_;
        pos_ctrl_status.xtrack_error = l1_crosstrack_error_;
        pos_ctrl_status.wp_dist = get_distance_to_next_waypoint(curr_pos_(1), curr_pos_(2), ...
        curr_wp_(1), curr_wp_(2));
        pos_ctrl_status.acceptance_radius = min(500, l1_distance_);
        pos_ctrl_status.yaw_acceptance = single(nan);
        settings: executionOrder=3
  (default) -> rotary_wing
  rotary_wing -> fixed_wing : [vehicle_status.vehicle_type ~= PX4_VEHICLE_STATUS.VEHICLE_TYPE_ROTARY_WING && ...
      | vehicle_status.in_transition_mode]
  fixed_wing -> rotary_wing : [vehicle_status.vehicle_type == PX4_VEHICLE_STATUS.VEHICLE_TYPE_ROTARY_WING && ...
      | ~vehicle_status.in_transition_mode]
  data: valid function_output; eas_to_tas function_output; man_sp_x function_output; man_sp_z function_output; state function_output; time_went_in_air_ local uint64 size=1 =uint64(0); z function_output; y function_output; x function_output; is_man_ctr function_output; nav_speed_2d function_output; ground_speed_2d function_output; alt function_output; position_sp_alt local single size=1; d_curr_prev local single size=1; d_curr local single size=1; min_current_sp_distance_xy_ local single size=1 =single(inf); loiter_type_ local; altitude_desired function_output; mode function_output; pitch_min_rad function_output; land_tecs_mode local Enum: PX4_TECS_STATUS size=1; wp_distance_ local single size=1 =single(0.0); bearing_lastwp_currwp_ local single size=1 =single(0.0); wp_distance_save local single size=1 =single(0.0); flare_length_ local single size=1 =single(0.0); H0_ local single size=1 =single(0.0); flare_constant_ local single size=1 =single(0.0); H1_virt local single size=1 =single(0.0); flare_curve_alt_rel local single size=1 =single(0.0); bearing_airplane_currwp_ local single size=1 =single(0.0); land_terrain_alt_ local single size=1 =single(0.0); motor_lim_relative_alt local single size=1 =single(0.0); flare_curve_alt_rel_last local single size=1 =single(0.0); flare_height local single size=1 =single(0.0); flare_pitch_sp local single size=1 =single(0.0); target_bearing_ local single size=1 =single(0.0); horizontal_slope_displacement_ local single size=1 =single(0.0); land_climbout_pitch_min_rad local single size=1; terrain_alt function_output; aspd function_output; alt function_output; alt function_input; takeoff_init_yaw_ local single size=1; takeoff_initialized_time_ local uint64 size=1; ramp_time_ local uint64 size=1; airspeed local single size=1; alt_agl local single size=1; start_wp_ local double size=[1 2]; takeoff_climbout_ local boolean size=1; takeoff_terrain_alt_ local single size=1; takeoff_pitch_max_deg_ local single size=1; takeoff_roll_body_ local single size=1; takeoff_yaw_body_ local single size=1; takeoff_initialized_ local boolean size=1; acc_rad local single size=1 =single(0); transition_wp_ local double size=[1 2] =[nan, nan]; mission_airspeed_ local single size=1; mission_throttle_ local single size=1; airspeed_demand_ local single size=1 =single(0.0); dist_xy local single size=1 =single(-1.0); dist_z local single size=1 =single(-1.0); dist local single size=1 =single(0.0); alt function_input; hdg_hold_yaw local size=1; yaw_lock_engaged_ local boolean size=1 =false; yawrate_ local size=1; hdg_hold_enabled_ local boolean size=1 =false; hdg_hold_prev_wp local size=[1 3] =; hdg_hold_curr_wp local size=[1 3] =; pos_mode_hold_alt_ local single size=1; pos_mode_pitch_limited_min_ local single size=1; pos_mode_throttle_max_ local single size=1; pos_mode_altctrl_airspeed local single size=1; pos_mode_desire_alt local single size=1; vector_A function_input double size=[1 2]; vector_B function_input double size=[1 2]; vector_curr_position function_input double size=[1 2]; ground_speed_vector function_input single size=[1 2]; att_sp_roll_body function_input single size=1; roll_body function_output; nav_bearing function_output; target_braring function_output; crosstrack_error function_output; distance function_output; circle_mode function_output; roll_sp function_output; circle_mode function_output; navigation_heading function_input single size=1; current_heading function_input single size=1; ground_speed_vector function_input single size=[1 2]; l1_heading_dis function_output; att_sp_roll_body function_input single size=1; vector_A function_input double size=[1 2]; vector_curr_position function_input double size=[1 2]; loiter_direction function_input int8 size=1; ground_speed_vector function_input single size=[1 2]; roll_sp function_output; nav_bearing function_output; target_bearing function_output; distance function_output; radius function_input single size=1; circle_mode function_output; curr_circle_mode function_input boolean size=1; att_sp_roll_body function_input single size=1; throttle_sp function_output; pitch_sp function_output; hgt_rate_sp function_output; tecs_input function_input Bus: px4_tecs_input size=1; tecs_mode function_output; out function_output; run_tecs function_output; tecs_control function_output; alt_sp function_input; airspeed_sp function_input; pitch_min_rad function_input; pitch_max_rad function_input; tecs_throttle_min function_input; tecs_throttle_max function_input; tecs_throttle_cruise function_input; climbout_mode function_input; climbout_pitch_min_rad function_input; mode function_input; hgt_rate_sp function_input; alt_mode_altctrl_airspeed local single size=1; alt_mode_desire_alt local single size=1; alt_mode_alt_hold local single size=1; other_mode_alt_hold local single size=1; out function_output; hold_alt function_output; pitch_lim_min function_output; thr_max function_output; reinitialize_tecs_ local size=1 =false; tas_rate_filtered_ local single size=1 =single(0.0); tecs_height_error_gain_ local single size=1 =single(0.2); tecs_pitch_speed_weight_ local single size=1 =single(1.0); run_tecs_ local boolean size=1 =false; tecs_thr_min_ local single size=1 =single(0.0); tecs_thr_max_ local single size=1 =single(1.0); tecs_miss_thr_ local single size=1 =single(0.0); was_in_deadband local boolean size=1 =false; althold_epv local single size=1 =single(0.0); manual_height_rate_setpoint_m_s_ local single size=1 =single(nan); asp_after_transition local single size=1 =single(0.0); pos_control_mode_ local Enum: PX4_FW_CONTROL size=1; tecs_throttle_sp_ local single size=1 =single(0.0); tecs_pitch_sp_ local single size=1 =single(0.0); tecs_mode_ local Enum: PX4_TECS_STATUS size=1; tecs_hgt_rate_sp_ local single size=1; tecs_fw_thr_max local single size=1; tecs_fw_thr_min local single size=1 =single(0); tecs_fw_mission_throttle local single size=1 =single(0); aspd_demand function_output; aspd function_input; force function_input; in_takeoff_situation_ local boolean size=1 =false; takeoff_ground_alt_ local size=1; air_speed_2d_ local size=[1 2]; air_gnd_angle local size=1; current_alt_ local size=1; was_in_transition local boolean size=1 =false; landed_ local size=1; land_abort_ local boolean size=1 =false; current_lat_ local size=1; current_lon_ local size=1; roll_ local size=1; pitch_ local size=1; yaw_ local size=1; R_ local size=[3 3]; body_acc_ local size=[1 3]; body_vel_ local size=[1 3]; circle_mode_ local boolean size=1 =false; was_in_air_ local boolean size=1 =false; time_started_landing_ local uint64 size=1 =uint64(0); time_last_t_alt_ local uint64 size=1 =uint64(0); land_noreturn_horizontal_ local boolean size=1 =false; land_noreturn_vertical_ local boolean size=1 =false; land_stayonground_ local boolean size=1 =false; land_motor_lim_ local boolean size=1 =false; land_onslope_ local boolean size=1 =false; launch_detection_state local size=1; run_way_takeoff_initialized local boolean size=1 =false; run_way_takeoff_state local size=1; is_tecs_running local boolean size=1; tecs_input_ local Bus: px4_tecs_input size=1; was_circle_mode_ local boolean size=1 =false; curr_pos_ local double size=[1 2]; curr_wp_ local double size=[1 2]; prev_wp_ local double size=[1 2]; pos_sp_prev_ local Bus: px4_position_setpoint size=1; pos_sp_curr_ local Bus: px4_position_setpoint size=1; pos_sp_next_ local Bus: px4_position_setpoint size=1; airspeed_valid_ local boolean size=1 =true; airspeed_valid_time local uint64 size=1 =uint64(0); eas2tas_ local single size=1 =single(1.0); man_ctr_sp_aspd_ local single size=1 =single(0.0); man_ctr_sp_alt_ local single size=1 =single(0.0); last_manual_ local boolean size=1 =false; nav_speed_2d_ local single size=[1 2]; ground_speed_2d_ local single size=[1 2]; throttle_max_ local single size=1 =single(1.0); l1_target_bearing_ local single size=1; l1_crosstrack_error_ local single size=1; l1_distance_ local single size=1 =single(20.0); curr_wp_type_ local uint8 size=1 =uint8(0); control_mode input; local_pos input; pos_sp_triplet input; vehicle_att input; vehicle_att_sp input; global_pos input; airspeed_validated input; vehicle_status input; vehicle_ang_vel input; man_ctr_sp input; land_detected input; HDG_HOLD_DIST_NEXT parameter; FW_THR_MIN parameter; FW_THR_MAX parameter; FW_CLMBOUT_DIFF parameter; FW_AIRSPD_MIN parameter; FW_PSP_OFF parameter; FW_LND_EARLYCFG parameter; FW_ARSP_MODE parameter; VT_ARSP_TRANS parameter; FW_AIRSPD_MAX parameter; FW_GND_SPD_MIN parameter; DT_DEFAULT parameter; FW_P_LIM_MIN parameter; FW_P_LIM_MAX parameter; FW_T_TAS_R_TC parameter; FW_T_CLMB_R_SP parameter; FW_T_SINK_R_SP parameter; FW_LND_AIRSPD_SC parameter; FW_LND_HHDIST parameter; FW_LND_FLALT parameter; FW_THR_LND_MAX parameter; FW_LND_TLALT parameter; FW_LND_ANG parameter; FW_LND_HVIRT parameter; FW_LND_FL_PMIN parameter; FW_AIRSPD_TRIM parameter; FW_THR_CRUISE parameter; FW_MAN_R_MAX parameter; FW_POSCTL_INV_ST parameter; ALTHOLD_EPV_RESET_THRESH parameter; RWTO_RAMP_TIME parameter; RWTO_AIRSPD_SCL parameter; RWTO_PSP parameter; FW_T_SPDWEIGHT parameter; FW_T_ALT_TC parameter; RWTO_TKOFF parameter; RWTO_HDG parameter; out_att_sp output Bus: px4_vehicle_attitude_setpoint; FW_LND_THRTC_SC parameter; FW_TKO_PITCH_MIN parameter; RWTO_MAX_PITCH parameter; RWTO_MAX_THR parameter; pos_ctrl_status output Bus: px4_position_controller_status; RWTO_MAX_ROLL parameter
  function define_variables:
    | function define_variables()
    | 
    | out_att_sp   = vehicle_att_sp;
    | 
    | landed_      = land_detected.landed;
    | 
    | % 当前纬度、经度、高度
    | current_lat_ = global_pos.lat;
    | current_lon_ = global_pos.lon;
    | current_alt_ = -local_pos.z + local_pos.ref_alt;
    | 
    | % 当前航点、上个航点、下个航点
    | curr_wp_     = [pos_sp_triplet.current.lat, pos_sp_triplet.current.lon];
    | prev_wp_     = [pos_sp_triplet.previous.lat, pos_sp_triplet.previous.lon];
    | curr_pos_    = [global_pos.lat, global_pos.lon];
    | 
    | % 航点数据
    | pos_sp_prev_ = pos_sp_triplet.previous;
    | pos_sp_curr_ = pos_sp_triplet.current;
    | pos_sp_next_ = pos_sp_triplet.next;
    | 
    | end
  function [valid, eas_to_tas] = airspeed_poll:
    | function [valid, eas_to_tas] = airspeed_poll()
    | 
    | % this is the default value, taken in case of invalid airspeed
    | persistent airspeed_valid_time;
    | 
    | valid = false;
    | eas_to_tas = single(1.0);
    | 
    | if (FW_ARSP_MODE == single(0)) && ...
    |         (isfinite(airspeed_validated.calibrated_airspeed_m_s) && ...
    |         (isfinite(airspeed_validated.true_airspeed_m_s)) && ...
    |         (airspeed_validated.calibrated_airspeed_m_s > single(0.0)))
    |     
    |     valid = true;
    |     eas_to_tas = constrain(airspeed_validated.true_airspeed_m_s / airspeed_validated.calibrated_airspeed_m_s, 0.9, 2.0);
    |     airspeed_valid_time = uint64(getSimulationTime);
    |     
    | elseif(uint64(getSimulationTime) * 1000 - airspeed_valid_time > 1000) % 空速计数据持续1s无效
    |     
    |     valid = false;
    |     airspeed_valid_time = uint64(0);
    |     
    | end
    | 
    | end
  function [man_sp_x, man_sp_z] = manual_control_setpoint_poll:
    | function [man_sp_x, man_sp_z] = manual_control_setpoint_poll()
    | 
    | man_sp_x = man_ctr_sp.x;
    | man_sp_z = constrain(man_ctr_sp.z, 0.0, 1.0);
    | 
    | % FW_POSCTL_INV_ST, default 0
    | % @value 0 Normal stick configuration (airspeed on throttle stick, altitude on pitch stick)
    | % @value 1 Alternative stick configuration (altitude on throttle stick, airspeed on pitch stick)
    | % value 0 油门控空速，俯仰控高度，默认方式
    | % value 1 可选配置，油门控高度，俯仰控空速
    | if(FW_POSCTL_INV_ST)
    |     man_sp_x = -single(constrain(man_ctr_sp.z, 0.0, 1.0) * 2.0 - 1.0);
    |     man_sp_z =  single(constrain(man_ctr_sp.x, -1.0, 1.0) / 2.0 + 0.5);
    | end
    | 
    | end
  function state = is_takeoff_situation:
    | % check if we are in a takeoff situation
    | function state = is_takeoff_situation
    | 
    | if (vehicle_status.is_vtol)
    |     state = false;
    | elseif ((uint64(getSimulationTime) * 1000 - time_went_in_air_ < 10000) && (current_alt_ <= (takeoff_ground_alt_ + FW_CLMBOUT_DIFF)))
    |     state = true;
    | else
    |     state = false;
    | end
    | 
    | end
  function [z, y, x] = vehicle_attitude_poll:
    | function [z, y, x] = vehicle_attitude_poll()
    | 
    | R_ = quat_to_dcm(vehicle_att.q);
    | [z, y, x] = dcm_to_euler(R_);
    | 
    | yawrate_ = vehicle_ang_vel.xyz(3);
    | 
    | body_acc_ = transpose(R_' * [local_pos.ax; local_pos.ay; local_pos.az]);
    | body_vel_ = transpose(R_' * [local_pos.vx; local_pos.vy; local_pos.vz]);
    | 
    | end
  function is_man_ctr = vehicle_control_mode_poll:
    | function is_man_ctr = vehicle_control_mode_poll()
    | 
    | persistent was_armed;
    | was_armed = control_mode.flag_armed;
    | 
    | % reset state when arming
    | % 刚解锁的时候重置起飞和降落的相关状态
    | if (~was_armed && control_mode.flag_armed)
    |     reset_takeoff_state(true);
    |     reset_landing_state();
    | end
    | 
    | if (control_mode.flag_control_position_enabled)
    |     is_man_ctr = false;
    | else
    |     is_man_ctr = true;
    | end
    | 
    | end
  function [nav_speed_2d, ground_speed_2d] = vehicle_update_nav_speed:
    | function [nav_speed_2d, ground_speed_2d] = vehicle_update_nav_speed()
    | 
    | ground_speed_2d = [local_pos.vx, local_pos.vy];
    | nav_speed_2d = ground_speed_2d;
    | 
    | if (airspeed_valid_)
    |     % l1 navigation logic breaks down when wind speed exceeds max airspeed
    |     % compute 2d groundspeed from airspeed-heading projection
    |     air_speed_2d_ = [airspeed_validated.calibrated_airspeed_m_s * cos(yaw_), airspeed_validated.calibrated_airspeed_m_s * sin(yaw_)];
    |     nav_speed_2d = [local_pos.vx, local_pos.vy];
    |     
    |     % angle between air_speed_2d_ and ground_speed
    |     air_gnd_angle = acos(dot(air_speed_2d_, nav_speed_2d) / norm(air_speed_2d_) * norm(nav_speed_2d));
    |     
    |     % if angle > 90 degrees or groundspeed is less than threshold, replace groundspeed with airspeed projection
    |     if ((abs(air_gnd_angle) > single(pi/2)) || (norm(nav_speed_2d) < single(3.0)))
    |         nav_speed_2d = air_speed_2d_;
    |     end
    | end
    | 
    | end
  function is_transition_to_fw:
    | % Autonomous Flight
    | function is_transition_to_fw
    | 
    | %% 过渡过程
    | if (vehicle_status.is_vtol && vehicle_status.in_transition_to_fw)
    |     
    |     if (~isfinite(transition_wp_(1)))
    |         % create a virtual waypoint HDG_HOLD_DIST_NEXT meters in front of the vehicle which the L1 controller can track
    |         % during the transition
    |         [transition_wp_(1), transition_wp_(2)] = waypoint_from_heading_and_distance(current_lat_, current_lon_, yaw_, HDG_HOLD_DIST_NEXT);
    |         curr_wp_  = transition_wp_;
    |         prev_wp_ = transition_wp_;
    |     else
    |         % current waypoint (the one currently heading for)
    |         if (pos_sp_prev_.valid)
    |             prev_wp_(1) = pos_sp_prev_.lat;
    |             prev_wp_(2) = pos_sp_prev_.lon;
    |         else
    |             % No valid previous waypoint, go for the current wp.
    |             % This is automatically handled by the L1 library.
    |             prev_wp_(1) = pos_sp_curr_.lat;
    |             prev_wp_(2) = pos_sp_curr_.lon;
    |         end
    |         
    |         % reset transition waypoint, will be set upon entering front transition
    |         transition_wp_ = [nan, nan];
    |     end
    |     
    | end
    | 
    | % reset hold altitude
    | hold_alt = current_alt_;
    | 
    | % reset hold yaw
    | hdg_hold_yaw = yaw_;
    | 
    | % get circle mode
    | was_circle_mode_ = circle_mode_;
    | 
    | % restore TECS parameters, in case changed intermittently (e.g. in landing handling)
    | tecs_pitch_speed_weight_ = single(FW_T_SPDWEIGHT);
    | tecs_height_error_gain_  = single(1.0 / max(FW_T_ALT_TC, 0.1));
    | 
    | % Initialize attitude controller integrator reset flags to 0
    | out_att_sp.roll_reset_integral  = false;
    | out_att_sp.pitch_reset_integral = false;
    | out_att_sp.yaw_reset_integral   = false;
    | 
    | % update mission_airspeed_
    | if(isfinite(pos_sp_curr_.cruising_speed) && (pos_sp_curr_.cruising_speed >= 0.1))
    |     mission_airspeed_ = pos_sp_curr_.cruising_speed;
    | else
    |     mission_airspeed_ = single(FW_AIRSPD_TRIM);
    | end
    | 
    | % update mission_throttle
    | if(isfinite(pos_sp_curr_.cruising_throttle) && (pos_sp_curr_.cruising_throttle >= 0.0))
    |     mission_throttle_ = pos_sp_curr_.cruising_throttle;
    | else
    |     mission_throttle_ = single(FW_THR_CRUISE);
    | end
    | 
    | if (mission_throttle_ < FW_THR_MIN)
    |     % 使用此航路点启用滑行
    |     tecs_pitch_speed_weight_ = single(2.0);
    |     tecs_thr_min_            = single(0.0);
    |     tecs_thr_max_            = single(0.0);
    |     tecs_miss_thr_           = single(0.0);
    | else
    |     tecs_pitch_speed_weight_ = single(FW_T_SPDWEIGHT);
    |     tecs_thr_min_            = single(FW_THR_MIN);
    |     tecs_thr_max_            = single(FW_THR_MAX);
    |     tecs_miss_thr_           = single(mission_throttle_);
    | end
    | 
    | % acceptance_radius 切换到下一个航点的最佳距离
    | acc_rad = min(single(500.0), l1_distance_);
    | 
    | end
  function alt = get_foh_alt:
    | function alt = get_foh_alt()
    | 
    |     % waypoint is a plain navigation waypoint
    |     alt = pos_sp_curr_.alt;
    | 
    |     % Altitude first order hold (FOH)
    |     if ((pos_sp_triplet.previous.valid) && ...
    |        ((pos_sp_triplet.previous.type == PX4_POSITION_SETPOINT.SETPOINT_TYPE_POSITION) || ...
    |         (pos_sp_triplet.previous.type == PX4_POSITION_SETPOINT.SETPOINT_TYPE_LOITER)   || ...
    |         (pos_sp_triplet.previous.type == PX4_POSITION_SETPOINT.SETPOINT_TYPE_TAKEOFF)))
    | 
    |         d_curr_prev = get_distance_to_next_waypoint(curr_wp_(1), curr_wp_(2), prev_wp_(1), prev_wp_(2));
    | 
    |         % Do not try to find a solution if the last waypoint is inside the acceptance radius of the current one
    |         if (d_curr_prev > max(acc_rad, abs(pos_sp_triplet.current.loiter_radius)))
    | 
    |             % Calculate distance to current waypoint
    |             d_curr = get_distance_to_next_waypoint(curr_wp_(1), curr_wp_(2), curr_pos_(1), curr_pos_(2));
    | 
    |             % Save distance to waypoint if it is the smallest ever achieved, however make sure that
    |             % _min_current_sp_distance_xy_ is never larger than the distance between the current and the previous wp
    |             min_current_sp_distance_xy_ = min([d_curr, min_current_sp_distance_xy_, d_curr_prev]);
    | 
    |             % if the minimal distance is smaller than the acceptance radius, we should be at waypoint alt
    |             % navigator will soon switch to the next waypoint item (if there is one) as soon as we reach this altitude
    |             if (min_current_sp_distance_xy_ > max(acc_rad, abs(pos_sp_triplet.current.loiter_radius)))
    | 
    |                 % The setpoint is set linearly and such that the system reaches the current altitude at the acceptance
    |                 % radius around the current waypoint
    |                 delta_alt = (pos_sp_triplet.current.alt - pos_sp_triplet.previous.alt);
    |                 grad = -delta_alt / (d_curr_prev - max(acc_rad, abs(pos_sp_triplet.current.loiter_radius)));
    |                 a = pos_sp_triplet.previous.alt - grad * d_curr_prev;
    | 
    |                 alt = single(a + grad * min_current_sp_distance_xy_);
    |             end
    | 
    |         end
    | 
    |     end
    | 
    | end
  function control_landing:
    | function control_landing
    | 
    | %% landing slope param update
    | % check if negative value for 2/3 of flare altitude is set for throttle cut
    | land_thrust_lim_alt_relative = single(FW_LND_TLALT);    % 推力限制高度，默认-1
    | 
    | if (FW_THR_LND_MAX > 0.0)
    |     land_thrust_lim_alt_relative = single(FW_THR_LND_MAX);
    | else
    |     land_thrust_lim_alt_relative = single(2/3 * FW_LND_FLALT);
    | end
    | 
    | % local variable
    | landing_slope_angle_rad = deg2rad(FW_LND_ANG);          % 默认下滑角，5度
    | flare_relative_alt = FW_LND_FLALT;                      % 默认拉平相对高度(relative to landing altitude):3m
    | motor_lim_relative_alt = land_thrust_lim_alt_relative;  % 在拉平过程中，低于这个高度就会油门限制，刚拉平的时候，该值为1，实际上这个高度应该是个比值
    | H1_virt = single(FW_LND_HVIRT);                         % 默认虚拟地下高度，10m
    | 
    | % global variable
    | H0_                             = single(flare_relative_alt + H1_virt);
    | d1                              = single(flare_relative_alt / tan(landing_slope_angle_rad));
    | flare_constant_                 = single((H0_ * d1) / flare_relative_alt);
    | flare_length_                   = single(-log(H1_virt / H0_) * flare_constant_);
    | horizontal_slope_displacement_  = single(flare_length_ - d1);
    | 
    | %% 准备参数
    | if (pos_sp_triplet.previous.valid)
    |     prev_wp_(1) = pos_sp_prev_.lat;
    |     prev_wp_(2) = pos_sp_prev_.lon;
    | else
    |     % No valid previous waypoint, go for the current wp. This is automatically handled by the L1 library.
    |     prev_wp_(1) = pos_sp_curr_.lat;
    |     prev_wp_(2) = pos_sp_curr_.lon;
    | end
    | 
    | % Enable tighter altitude control for landings
    | tecs_height_error_gain_ = single(FW_LND_THRTC_SC * FW_T_ALT_TC);
    | 
    | bearing_airplane_currwp_ = get_bearing_to_next_waypoint(curr_pos_(1), curr_pos_(2), curr_wp_(1), curr_wp_(2));
    | bearing_lastwp_currwp_   = get_bearing_to_next_waypoint(prev_wp_(1), prev_wp_(2), curr_wp_(1), curr_wp_(2));
    | 
    | %% Horizontal landing control
    | % switch to heading hold for the last meters, continue heading hold after
    | wp_distance_ = get_distance_to_next_waypoint(curr_pos_(1), curr_pos_(2), curr_wp_(1), curr_wp_(2));
    | 
    | % calculate a waypoint distance value which is 0 when the aircraft is behind the waypoint
    | delta_bearing = abs(wrap((bearing_airplane_currwp_ - bearing_lastwp_currwp_), -pi, pi));
    | 
    | if (delta_bearing >= deg2rad(90.0))
    |     wp_distance_save = single(0.0);
    | else
    |     wp_distance_save = single(wp_distance_);
    | end
    | 
    | % create virtual waypoint which is on the desired flight path but
    | % some distance behind landing waypoint. This will make sure that the plane
    | % will always follow the desired flight path even if we get close or past
    | % the landing waypoint
    | if (pos_sp_prev_.valid)
    |     [curr_wp_(1), curr_wp_(2)] = create_waypoint_from_line_and_dist(pos_sp_curr_.lat, pos_sp_curr_.lon, ...
    |         pos_sp_prev_.lat, pos_sp_prev_.lon, -1000.0);
    | end
    | 
    | end
  function altitude_desired = glide_slope:
    | % intersect glide slope:
    | % minimize speed to approach speed
    | % if current position is higher than the slope follow the glide slope (sink to the glide slope)
    | % also if the system captures the slope it should stay
    | % on the slope (bool land_onslope_)
    | % if current position is below the slope continue at previous wp altitude
    | % until the intersection with slope
    | 
    | function altitude_desired = glide_slope
    | 
    | altitude_desired = land_terrain_alt_;
    | 
    | % getLandingSlopeRelativeAltitudeSave
    | % If airplane is in front of waypoint return flare curve altitude, else return waypoint altitude
    | if (abs(wrap(bearing_airplane_currwp_ - bearing_lastwp_currwp_, -pi, pi)) < deg2rad(90.0))
    |     % 飞机还没有飞过当前的航点
    |     temp = -max(0.0, (flare_length_ - wp_distance_) / flare_constant_) - H1_virt;
    |     LandingSlopeRelativeAltitudeSave = (H0_ * exp(1)^temp);
    | else
    |     LandingSlopeRelativeAltitudeSave = single(0.0);
    | end
    | 
    | landing_slope_alt_rel_desired = LandingSlopeRelativeAltitudeSave;
    | 
    | if (current_alt_ > land_terrain_alt_ + landing_slope_alt_rel_desired)
    |     % stay on slope
    |     altitude_desired = land_terrain_alt_ + landing_slope_alt_rel_desired;
    | else
    |     % continue horizontally, 当前高度低于期望高度，保持当前高度，直到能满足slope angle的时候
    |     if (pos_sp_prev_.valid)
    |         altitude_desired = pos_sp_prev_.alt;
    |     else
    |         altitude_desired = current_alt_;
    |     end
    | end
    | 
    | end
  function [mode, pitch_min_rad] = start_flaring:
    | function [mode, pitch_min_rad] = start_flaring
    | 
    | % Only kill throttle when close to WP
    | % FW_THR_MAX最大油门百分比 默认：1.0
    | throttle_max_ = single(FW_THR_MAX);
    | 
    | % 进入预设的水平距离以后，允许直接控制方向舵或轮胎
    | if (land_noreturn_horizontal_)
    |     out_att_sp.yaw_body = target_bearing_;
    |     out_att_sp.fw_control_yaw = true;
    | end
    | 
    | % Only kill throttle when close to WP
    | if ((current_alt_ < land_terrain_alt_ + motor_lim_relative_alt) && (wp_distance_save < flare_length_ + 5.0) || ...
    |         land_motor_lim_)
    |     throttle_max_ = min(throttle_max_, FW_THR_LND_MAX);
    |     land_motor_lim_ = true;
    | end
    | 
    | % If airplane is in front of waypoint return flare curve altitude, else return waypoint altitude */
    | if (abs(wrap(bearing_airplane_currwp_ - bearing_lastwp_currwp_, -pi, pi)) < deg2rad(90.0))
    |     flare_curve_alt_rel = single(H0_ * exp(-max(0.0, flare_length_ - wp_distance_) / flare_constant_) - H1_virt);
    | else
    |     flare_curve_alt_rel = single(0.0);
    | end
    | 
    | % avoid climbout
    | if (flare_curve_alt_rel_last < flare_curve_alt_rel && land_noreturn_vertical_)
    |     flare_curve_alt_rel = single(0.0); % stay on ground
    | end
    | 
    | airspeed_land = single(FW_LND_AIRSPD_SC * FW_AIRSPD_MIN);
    | throttle_land = single(FW_THR_MIN + (FW_THR_MAX - FW_THR_MIN) * 0.1);
    | 
    | airspeed_demand_ = cal_target_aspd(airspeed_land);
    | 
    | if (land_motor_lim_)
    |     pitch_min_rad = single(deg2rad(FW_LND_FL_PMIN));
    |     mode = PX4_TECS_STATUS.TECS_MODE_LAND_THROTTLELIM;
    |     
    | else
    |     pitch_min_rad = single(deg2rad(FW_P_LIM_MIN));
    |     mode = PX4_TECS_STATUS.TECS_MODE_LAND;
    | end
    | 
    | end
  function takeoff_init:
    | % run takeoff state init
    | function takeoff_init
    | 
    | takeoff_init_yaw_ = yaw_;
    | takeoff_initialized_ = true;
    | takeoff_initialized_time_ = uint64(getSimulationTime);
    | takeoff_climbout_ = true;                       % this is true until climbout is finished
    | start_wp_ = [current_lat_, current_lon_];
    | takeoff_ground_alt_ = current_alt_;              % 绝对海平面高度，单位：m
    | 
    | end
  function terrain_alt = get_terrain_altitude_takeoff:
    | % 在起飞或降落时返回地形估计
    | function terrain_alt = get_terrain_altitude_takeoff
    | 
    | if (pos_sp_prev_.valid)
    |     prev_wp_(1) = pos_sp_prev_.lat;
    |     prev_wp_(2) = pos_sp_prev_.lon;
    | else
    |     % No valid previous waypoint, go for the current wp.
    |     % This is automatically handled by the L1 library.
    |     prev_wp_(1) = pos_sp_curr_.lat;
    |     prev_wp_(2) = pos_sp_curr_.lon;
    | end
    | 
    | % continuously reset launch detection and runway takeoff until armed
    | if (control_mode.flag_armed)
    |     takeoff_initialized_ = false;
    |     launch_detection_state = PX4_LAUNCH_DETECTION_RESULT.LAUNCHDETECTION_RES_NONE;
    | end
    | 
    | % 当地的海平面高度(地形高度WGS84(米)) = 参考海平面高度 - （Distance from from bottom surface to ground + Down
    | % position (negative altitude) in NED earth - fixed frame） 单位：m
    | temp_alt = local_pos.ref_alt - (local_pos.dist_bottom + local_pos.z);
    | 
    | if (isfinite(temp_alt) && local_pos.dist_bottom_valid)
    |     terrain_alt = temp_alt;
    | else
    |     terrain_alt = takeoff_ground_alt_;
    | end
    | 
    | end
  function [aspd, alt] = cal_airspeed_alt(alt):
    | function [aspd, alt] = cal_airspeed_alt(alt)
    | 
    | % prepare data for update runway takeoff helper
    | aspd = airspeed_validated.calibrated_airspeed_m_s;
    | alt = current_alt_ - takeoff_terrain_alt_;
    | current_lat_ = pos_sp_curr_.lat;
    | current_lon_ = pos_sp_curr_.lon;
    | 
    | end
  function heading_control(alt):
    | % heading control
    | function heading_control(alt)
    | 
    | HDG_HOLD_MAN_INPUT_THRESH = single(0.01);
    | HDG_HOLD_YAWRATE_THRESH = single(0.15);
    | HDG_HOLD_REACHED_DIST =	single(1000.0);   % distance (plane to waypoint in front) at which waypoints are reset in heading hold mode
    | 
    | yawrate_ = vehicle_ang_vel.xyz(3);
    | hdg_hold_curr_wp = [0, 0, 0];
    | hdg_hold_prev_wp = [0, 0, 0];
    | 
    | if (abs(man_ctr_sp.y) < HDG_HOLD_MAN_INPUT_THRESH && abs(man_ctr_sp.r) < HDG_HOLD_MAN_INPUT_THRESH)
    |     
    |     % heading / roll is zero, lock onto current heading
    |     if (abs(yawrate_) < HDG_HOLD_YAWRATE_THRESH && ~yaw_lock_engaged_)
    |         % little yaw movement, lock to current heading
    |         yaw_lock_engaged_ = true;
    |     end
    |     
    |     % user tries to do a takeoff in heading hold mode, reset the yaw setpoint on every iteration
    |     % to make sure the plane does not start rolling
    |     % 用户起飞阶段锁定航向
    |     if (in_takeoff_situation_)
    |         hdg_hold_enabled_ = false;
    |         yaw_lock_engaged_ = true;
    |     end
    |     
    |     % if (yaw_lock_engaged_)
    |     % just switched back from non heading-hold to heading hold
    |     % 航向没锁定 ----> 航向锁定时才运行
    |     % hdg_holdyaw 航向锁定时的角度
    |     if (~hdg_hold_enabled_)
    |         hdg_hold_enabled_ = true;
    |         hdg_hold_yaw = yaw_;
    |         [hdg_hold_prev_wp, hdg_hold_curr_wp] = get_waypoint_heading_distance(hdg_hold_yaw, hdg_hold_prev_wp, hdg_hold_curr_wp, curr_pos_, alt, true);
    |     end
    |     
    |     % we have a valid heading hold position, are we too close?
    |     % 如果飞机与当前航点的距离小于1000米，重新计算当前的航点
    |     dist = get_distance_to_next_waypoint(curr_pos_(1), curr_pos_(2), hdg_hold_curr_wp(1), hdg_hold_curr_wp(2));
    |     
    |     if (dist < HDG_HOLD_REACHED_DIST)
    |         hdg_hold_curr_wp = get_waypoint_heading_distance(hdg_hold_yaw, hdg_hold_prev_wp, hdg_hold_curr_wp, curr_pos_, alt, false);
    |     end
    |     
    |     prev_wp = [hdg_hold_prev_wp(1), hdg_hold_prev_wp(2)];
    |     curr_wp = [hdg_hold_curr_wp(1), hdg_hold_curr_wp(2)];
    |     
    |     [out_att_sp.roll_body, out_att_sp.yaw_body, ...
    |         l1_target_bearing_, l1_crosstrack_error_, ...
    |         l1_distance_, circle_mode_] = ...
    |         l1_navigate_waypoints(prev_wp_, curr_wp_, curr_pos_, nav_speed_2d_, out_att_sp.roll_body);
    |     
    |     if (in_takeoff_situation_)
    |         % limit roll motion to ensure enough lift
    |         out_att_sp.roll_body = constrain(out_att_sp.roll_body, deg2rad(-15.0), deg2rad(15.0));
    |     end
    |     
    | end
    | 
    | if (~yaw_lock_engaged_ || abs(man_ctr_sp.y) >= HDG_HOLD_MAN_INPUT_THRESH || abs(man_ctr_sp.r) >= HDG_HOLD_MAN_INPUT_THRESH)
    |     hdg_hold_enabled_ = false;
    |     yaw_lock_engaged_ = false;
    |     out_att_sp.roll_body = single(man_ctr_sp.y * deg2rad(FW_MAN_R_MAX));
    |     out_att_sp.yaw_body = single(0.0);
    | end
    | 
    | end
  function out = get_demanded_airspeed:
    | % update desired airspeed based on user pitch stick input
    | function out = get_demanded_airspeed
    | 
    | % neutral throttle corresponds to trim airspeed
    | if (man_ctr_sp_aspd_ < 0.5)
    |     % lower half of throttle is min to trim airspeed
    |     % 油门在中下对应配平空速
    |     out = FW_AIRSPD_MIN + (FW_AIRSPD_TRIM - FW_AIRSPD_MIN) * man_ctr_sp_aspd_ * 2.0;
    | else
    |     % upper half of throttle is trim to max airspeed
    |     out = FW_AIRSPD_TRIM + (FW_AIRSPD_MAX - FW_AIRSPD_TRIM) * (man_ctr_sp_aspd_ * 2.0 - 1.0);
    | end
    | 
    | end
  function [run_tecs, tecs_control] = prepare_tecs_controller_param(alt_sp, ...:
    | function [run_tecs, tecs_control] = prepare_tecs_controller_param(alt_sp, ...
    |     airspeed_sp, ...
    |     pitch_min_rad, ...
    |     pitch_max_rad, ...
    |     tecs_throttle_min, ...
    |     tecs_throttle_max, ...
    |     tecs_throttle_cruise, ...
    |     climbout_mode, ...
    |     climbout_pitch_min_rad, ...
    |     mode, ...
    |     hgt_rate_sp)
    | 
    | % do not run TECS if we are not in air
    | run_tecs = ~landed_;
    | 
    | % do not run TECS if vehicle is a VTOL and we are in rotary wing mode or in transition
    | % (it should also not run during VTOL blending because airspeed is too low still)
    | if (vehicle_status.is_vtol)
    |     
    |     if ((vehicle_status.vehicle_type == uint8(PX4_VEHICLE_STATUS.VEHICLE_TYPE_ROTARY_WING)) || ...
    |             vehicle_status.in_transition_mode)
    |         run_tecs = false;
    |     end
    |     
    |     if (vehicle_status.in_transition_mode)
    |         
    |         was_in_transition = true;
    |         % set this to transition airspeed to init tecs correctly
    |         % FW_ARSP_MODE 对于小机翼或VTOL,没有空速传感器,可以使用这个参数，在没有空速读数的情况下飞行
    |         % FW_ARSP_MODE: 1 disable airspeed
    |         % VT_ARSP_TRANS: Airspeed at which we can switch to fw mode 默认10m/s
    |         if ((FW_ARSP_MODE == 1) && (isfinite(VT_ARSP_TRANS)))
    |             asp_after_transition = single(VT_ARSP_TRANS);
    |         else
    |             % 有空速计且使能使用空速计的数据
    |             asp_after_transition = airspeed_validated.calibrated_airspeed_m_s;
    |         end
    |         
    |         asp_after_transition = constrain(asp_after_transition, FW_AIRSPD_MIN, FW_AIRSPD_MAX);
    |         
    |     elseif (was_in_transition)
    |         
    |         % after transition we ramp up desired airspeed from the speed we had coming out of the transition
    |         asp_after_transition = asp_after_transition + DT_DEFAULT * 2.0; % increase 2m/s
    |         
    |         if ((asp_after_transition < airspeed_sp) && (airspeed_validated.calibrated_airspeed_m_s < airspeed_sp))
    |             airspeed_sp = single(max(asp_after_transition, airspeed_validated.calibrated_airspeed_m_s));
    |         else
    |             was_in_transition = false;
    |             asp_after_transition = single(0.0);
    |         end
    |         
    |     end
    |     
    | end
    | 
    | % 记录当前时刻是否在运行tecs控制器
    | is_tecs_running = run_tecs;
    | 
    | if (~run_tecs)
    |     % next time we run TECS we should reinitialize states
    |     reinitialize_tecs_ = true;
    | end
    | 
    | if (reinitialize_tecs_)
    |     states_initialized  = false;
    |     reinitialize_tecs_  = false;
    | end
    | 
    | if (vehicle_status.engine_failure)
    |     % Force the slow downwards spiral
    |     pitch_min_rad = single(deg2rad(-1.0));
    |     pitch_max_rad = single(deg2rad(5.0));
    | end
    | 
    | % tell TECS to update its state, but let it know when it cannot actually control the plane
    | in_air_alt_control = (~landed_ && (control_mode.flag_control_auto_enabled || control_mode.flag_control_velocity_enabled || control_mode.flag_control_altitude_enabled));
    | 
    | % update TECS vehicle state estimates
    | tecs_update_vehicle_state_estimates(airspeed_validated.calibrated_airspeed_m_s, ...
    |     body_acc_(1), ...
    |     local_pos.timestamp > single(0.0), ...
    |     in_air_alt_control, ...
    |     current_alt_, ...
    |     local_pos.vz);
    | 
    | % input for tecs control
    | tecs_control.mode                   = uint8(mode);
    | tecs_control.in_air                 = boolean(in_air_alt_control);
    | tecs_control.euler                  = single([roll_, pitch_ - deg2rad(FW_PSP_OFF), yaw_]);
    | tecs_control.body_vel               = single(body_vel_);
    | tecs_control.baro_altitude          = single(current_alt_);
    | tecs_control.hgt_setpoint           = single(alt_sp);
    | tecs_control.EAS_setpoint           = single(airspeed_sp);
    | tecs_control.equivalent_airspeed    = single(airspeed_validated.calibrated_airspeed_m_s);
    | tecs_control.eas_to_tas             = single(eas2tas_);
    | tecs_control.climb_out_setpoint     = boolean(climbout_mode);
    | tecs_control.pitch_min_climbout     = single(climbout_pitch_min_rad - FW_PSP_OFF);
    | tecs_control.throttle_min           = single(tecs_throttle_min);
    | tecs_control.throttle_max           = single(tecs_throttle_max);
    | tecs_control.throttle_cruise        = single(tecs_throttle_cruise);
    | tecs_control.pitch_limit_min        = single(pitch_min_rad - FW_PSP_OFF);
    | tecs_control.pitch_limit_max        = single(pitch_max_rad - FW_PSP_OFF);
    | tecs_control.target_climbrate       = single(FW_T_CLMB_R_SP);
    | tecs_control.target_sinkrate        = single(FW_T_SINK_R_SP);
    | tecs_control.hgt_rate_sp            = single(hgt_rate_sp);
    | tecs_control.height_error_gain      = single(tecs_height_error_gain_);
    | tecs_control.local_pos_vz           = single(local_pos.vz);
    | tecs_control.pitch_speed_weight     = single(tecs_pitch_speed_weight_);
    | tecs_control.speed_deriv_forward    = single(body_acc_(1));
    | tecs_control.tas_rate_filtered      = single(tas_rate_filtered_);
    | 
    | end
    | 
    | 
    | % Updates the following vehicle kineamtic state estimates:
    | % Vertical position, velocity and acceleration.
    | % Speed derivative
    | % Must be called prior to udating tecs control loops
    | % Must be called at 50Hz or greater
    | function tecs_update_vehicle_state_estimates(equivalent_airspeed, speed_deriv_forward, ...
    |     altitude_lock, in_air, altitude, vz)
    | 
    | % Set the velocity and position state to the the INS data
    | vert_vel_state = -vz;
    | vert_pos_state = altitude;
    | 
    | % Update and average speed rate of change if airspeed is being measured
    | if (isfinite(equivalent_airspeed))
    |     tas_rate_raw = speed_deriv_forward;
    |     % Apply some noise filtering
    |     alpha = DT_DEFAULT / (DT_DEFAULT + FW_T_TAS_R_TC);
    |     tas_rate_filtered_ = (1.0 - alpha) * tas_rate_filtered_ + alpha * tas_rate_raw;
    | else
    |     tas_rate_raw = single(0.0);
    |     tas_rate_filtered_ = single(0.0);
    | end
    | 
    | end
  function out = update_desired_altitude:
    | % update desired altitude based on user pitch stick input
    | function out = update_desired_altitude
    | 
    | persistent last_out;
    | last_out = single(0.0);
    | 
    | out = current_alt_;
    | 
    | % The complete range is -1..+1, so this is 6%
    | % of the up or down range or 3% of the total range.
    | deadBand = single(0.06);
    | 
    | % The correct scaling of the complete range needs
    | % to account for the missing part of the slope
    | % due to the deadband
    | factor = 1.0 - deadBand;
    | 
    | % Reset the hold altitude to the current altitude if the uncertainty
    | % changes significantly.
    | % This is to guard against uncommanded altitude changes
    | % when the altitude certainty increases or decreases.
    | if (abs(althold_epv - local_pos.epv) > ALTHOLD_EPV_RESET_THRESH)
    |     out = current_alt_;
    |     althold_epv = local_pos.epv;
    | end
    | 
    | % Manual control has as convention the rotation around
    | % an axis. Positive X means to rotate positively around
    | % the X axis in NED frame, which is pitching down
    | if (man_ctr_sp_alt_ > deadBand)
    |     % pitching down
    |     pitch = -(man_ctr_sp_alt_ - deadBand) / factor;
    |     
    |     if (pitch_ * FW_T_SINK_R_SP < tecs_hgt_rate_sp_)
    |         out = out * (FW_T_SINK_R_SP * DT_DEFAULT) * pitch_;
    |         manual_height_rate_setpoint_m_s_ = single(pitch_ * FW_T_SINK_R_SP);
    |         was_in_deadband = false;
    |     end
    |     
    | elseif (man_ctr_sp_alt_ < -deadBand)
    |     % pitching up
    |     pitch_ = -(man_ctr_sp_alt_ + deadBand) / factor;
    |     
    |     if (pitch_ * FW_T_CLMB_R_SP > tecs_hgt_rate_sp_)
    |         out = last_out + FW_T_CLMB_R_SP * DT_DEFAULT * pitch_;
    |         manual_height_rate_setpoint_m_s_ = single(pitch_ * FW_T_CLMB_R_SP);
    |         was_in_deadband = false;
    |     end
    |     
    | elseif (~was_in_deadband)
    |     % store altitude at which manual.x was inside deadBand
    |     % The aircraft should immediately try to fly at this altitude
    |     % as this is what the pilot expects when he moves the stick to the center
    |     out = current_alt_;
    |     althold_epv = local_pos.epv;
    |     was_in_deadband = true;
    |     manual_height_rate_setpoint_m_s_ = single(nan);
    | end
    | 
    | if ((vehicle_status.is_vtol) && (vehicle_status.vehicle_type == PX4_VEHICLE_STATUS.VEHICLE_TYPE_ROTARY_WING || vehicle_status.in_transition_mode))
    |     out = current_alt_;
    | end
    | 
    | last_out = out;
    | 
    | end
  function [hold_alt, pitch_lim_min, thr_max] = do_takeoff_help:
    | % if we assume that user is taking off then help by demanding altitude setpoint well above ground
    | % and set limit to pitch angle to prevent steering into ground
    | % this will only affect planes and not VTOL
    | function [hold_alt, pitch_lim_min, thr_max] = do_takeoff_help
    | 
    | THROTTLE_THRESH = single(0.05);
    | pitch_lim_min = single(FW_P_LIM_MIN);
    | hold_alt = single(pos_sp_curr_.alt);
    | 
    | % demand "climbout_diff" m above ground if user switched into this mode during takeoff
    | if (in_takeoff_situation_)
    |     hold_alt = single(takeoff_ground_alt_ + FW_CLMBOUT_DIFF);
    |     pitch_lim_min = single(deg2rad(10.0));
    | end
    | 
    | % throttle limiting
    | % thr_max = single(1.0);
    | if (landed_ && (abs(man_ctr_sp_aspd_) < THROTTLE_THRESH))
    |     thr_max = single(0.0);
    | else
    |     thr_max = single(FW_THR_MAX);
    | end
    | 
    | end
  function aspd_demand  = cal_target_aspd(aspd):
    | % Calculate accelerated stall airspeed factor from commanded bank angle and use it to increase minimum airspeed.
    | %
    | % We don't know the stall speed of the aircraft, but assuming user defined
    | % minimum airspeed (FW_AIRSPD_MIN) is slightly larger than stall speed
    | % this is close enough.
    | %
    | % increase lift vector to balance additional weight in bank
    | % cos(bank angle) = W/L = 1/n
    | % n is the load factor
    | %
    | % lift is proportional to airspeed^2 so the increase in stall speed is
    | % Vsacc = Vs * sqrt(n)
    |   
    | function aspd_demand  = cal_target_aspd(aspd)
    | 
    |     if (isfinite(out_att_sp.roll_body))
    |         adjusted_min_airspeed = constrain(FW_AIRSPD_MIN / sqrt(cos(vehicle_att_sp.roll_body)), FW_AIRSPD_MIN, FW_AIRSPD_MAX);
    |     else
    |         adjusted_min_airspeed = FW_AIRSPD_MIN;
    |     end
    | 
    | 	% groundspeed undershoot
    | 	if (~circle_mode_)
    |         % This error value ensures that a plane (as long as its throttle capability is
    |         % not exceeded) travels towards a waypoint (and is not pushed more and more away
    |         % by wind). Not countering this would lead to a fly-away.
    | 
    |         % add minimum ground speed undershoot (only non-zero in presence of sufficient wind)
    |         if (body_vel_(1) < FW_GND_SPD_MIN)
    |              aspd = aspd + max(FW_GND_SPD_MIN - body_vel_(1), 0);
    |         end
    |         
    |     end
    |     
    | 	% sanity check: limit to range
    | 	aspd_demand = constrain(aspd, adjusted_min_airspeed, FW_AIRSPD_MAX);
    |     
    | end
  function reset_landing_state:
    | function reset_landing_state()
    | 
    | time_started_landing_ = uint64(0);
    | 
    | % reset terrain estimation relevant values
    | % 上次地形数据有效的时间
    | time_last_t_alt_ = uint64(0);
    | 
    | land_noreturn_horizontal_ = false;
    | land_noreturn_vertical_ = false;
    | land_stayonground_ = false;
    | land_motor_lim_ = false;
    | land_onslope_ = false;
    | 
    | % reset abort land, unless loitering after an abort
    | if (land_abort_ && (pos_sp_triplet.current.type ~= PX4_POSITION_SETPOINT.SETPOINT_TYPE_LOITER))
    |     land_abort_ = false;
    | end
    | 
    | end
  function reset_takeoff_state(force):
    | function reset_takeoff_state(force)
    | 
    | % only reset takeoff if !armed or just landed_
    | if (~control_mode.flag_armed || (was_in_air_ && landed_) || force)
    |     run_way_takeoff_initialized = false;
    |     run_way_takeoff_state = PX4_TAKEOFF_STAGE.THROTTLE_UP;
    |     % launchDetector.reset();
    | else
    |     launch_detection_state = PX4_LAUNCH_DETECTION_RESULT.LAUNCHDETECTION_RES_DETECTED_ENABLEMOTORS;
    | end
    | 
    | end
